simulink model "Free_Flight_PID_RPY_ARDrone_TrayZ"  (R2016b)
settings: configuration reference "AR_Drone_ConfigSet" (kept outside this file)
undefined symbols (not defined in the file): accelerometerXyzGains, accelerometerXyzOffsets, DiscIntNeverNeededParam, gyroXyzOffsets, Mag_Calib_Gain_Vector, Mag_Calib_Offset_Vector
libraries: simulink x6, AR_Drone_Sensors x2, AR_Drone_Actuators x2, vrlib x2, dspnetwork x1, simulink_extras x1, etargetslib x1
settings Model: DataDictionary=ArDroneDataDictionary.sldd  SimulationMode=external  ExtModeTrigDuration=48000  Creator=nraman  LastModifiedBy=SCBR
settings ConfigSetRef: DDName=ArDroneDataDictionary.sldd

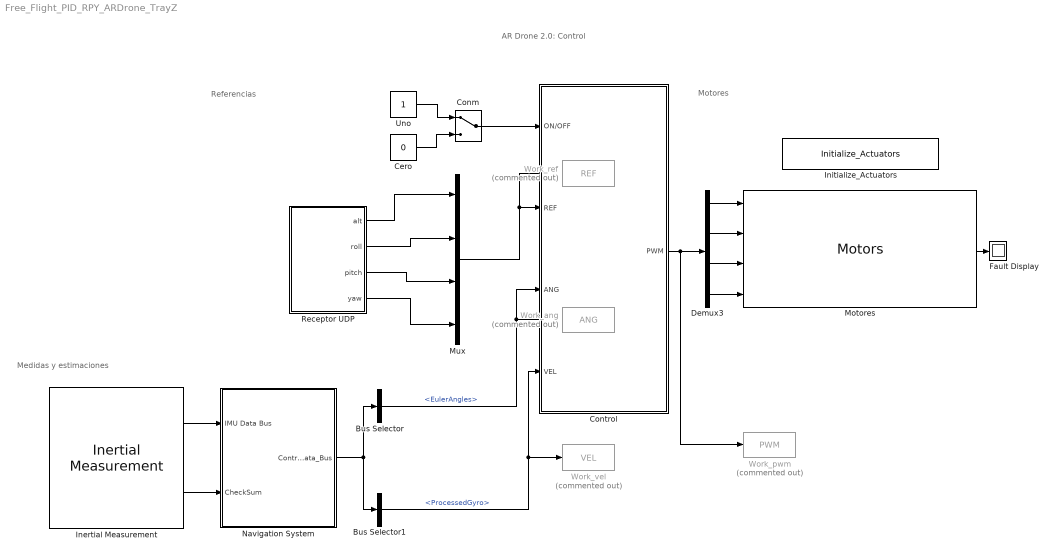
== system Free_Flight_PID_RPY_ARDrone_TrayZ ==
  note: AR Drone 2.0: Control
  note: Motores
  note: Medidas y estimaciones
  note: Referencias
  Bus Selector : BusSelector  OutputSignals=EulerAngles
  Bus Selector1 : BusSelector  OutputSignals=ProcessedGyro
  Cero : Constant  Value=0
  Conm : ManualSwitch
  Control : Subsystem
  Demux3 : Demux
  Fault Display : Display
  Inertial Measurement : AR_Drone_Sensors/Inertial Measurement  Ts=1/400
  Initialize_Actuators : AR_Drone_Actuators/Initialize_Actuators  ShowSpec=on
  Motores : AR_Drone_Actuators/Motors
  Mux : Mux
  Navigation System : Subsystem  AncestorBlock=AR_Drone_Positioning/Navigation System
  Receptor UDP : Subsystem
  Uno : Constant
  Work_ang : ToWorkspace  Commented=on  VariableName=ANG  SaveFormat=Structure With Time  SampleTime=0.0025
  Work_pwm : ToWorkspace  Commented=on  VariableName=PWM  SaveFormat=Structure With Time  SampleTime=0.0025
  Work_ref : ToWorkspace  Commented=on  VariableName=REF  SaveFormat=Structure With Time  SampleTime=0.0025
  Work_vel : ToWorkspace  Commented=on  VariableName=VEL  SaveFormat=Structure With Time  SampleTime=0.0025
  wires:
  Motores/1 -> Fault Display/1
  Demux3/1 -> Motores/1
  Demux3/2 -> Motores/2
  Demux3/3 -> Motores/3
  Demux3/4 -> Motores/4
  Inertial Measurement/1 -> Navigation System/1(IMU Data Bus)
  Inertial Measurement/2 -> Navigation System/2(CheckSum)
  Navigation System/1(Controller_Data_Bus) -> Bus Selector1/1, Bus Selector/1
  Bus Selector/1 -> Work_ang/1, Control/3(ANG)  "<EulerAngles>"
  Control/1(PWM) -> Work_pwm/1, Demux3/1
  Conm/1 -> Control/1(ON/OFF)
  Cero/1 -> Conm/2
  Uno/1 -> Conm/1
  Receptor UDP/1(alt) -> Mux/1
  Bus Selector1/1 -> Work_vel/1, Control/4(VEL)  "<ProcessedGyro>"
  Mux/1 -> Work_ref/1, Control/2(REF)
  Receptor UDP/2(roll) -> Mux/2
  Receptor UDP/3(pitch) -> Mux/3
  Receptor UDP/4(yaw) -> Mux/4

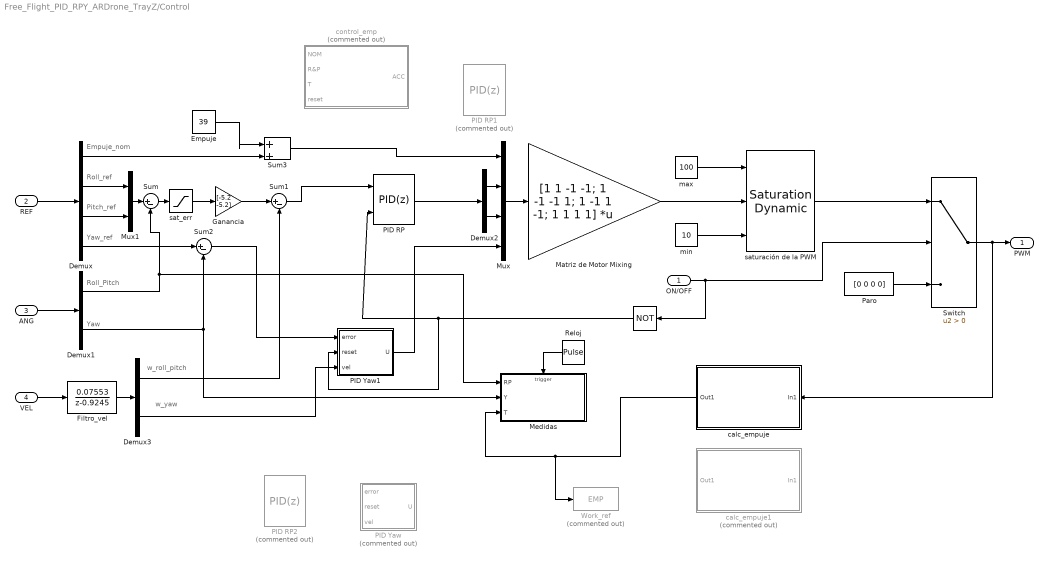
== system Free_Flight_PID_RPY_ARDrone_TrayZ/Control ==
  note: Empuje_nom
  note: Roll_ref
  note: Pitch_ref
  note: Yaw_ref
  note: Roll_Pitch
  note: Yaw
  note: w_roll_pitch
  note: w_yaw
  ON/OFF : Inport
  REF : Inport  Port=2
  ANG : Inport  Port=3
  VEL : Inport  Port=4
  " " : Logic  Operator=NOT  AllPortsSameDT=off  OutDataTypeStr=boolean
  Demux : Demux
  Demux1 : Demux  Outputs=[2 1]
  Demux2 : Demux  Outputs=2
  Demux3 : Demux  Outputs=[2 1]
  Empuje : Constant  Value=39
  Filtro_vel : DiscreteTransferFcn  Numerator=[0.07553]  Denominator=[1 -0.9245]
  Ganancia : Gain  Gain=[-5.2 -5.2]
  Matriz de Motor Mixing : Gain  Gain=[1 1 -1 -1; 1 -1 -1 1; 1 -1 1 -1; 1 1 1 1]  Multiplication=Matrix(K*u)  ParamDataTypeStr=int16  OutDataTypeStr=int16
  Medidas : Subsystem
  Mux : Mux
  Mux1 : Mux  Inputs=2
  PID RP : simulink/Continuous/PID Controller  Controller=PID  TimeDomain=Discrete-time  SampleTime=-1  IntegratorMethod=Forward Euler  FilterMethod=Forward Euler  Form=Parallel  UseFilter=on  ControllerParametersSource=internal  P=0.5  I=0.3  D=-0.04  N=5  InitialConditionSource=internal  InitialConditionForIntegrator=0  InitialConditionForFilter=0  ExternalReset=level  LimitOutput=on  UpperSaturationLimit=30  LowerSaturationLimit=-30  LinearizeAsGain=on  AntiWindupMode=clamping  Kb=1  TrackingMode=off  Kt=1  PParamMin=[]  PParamMax=[]  IParamMin=[]  IParamMax=[]  DParamMin=[]  DParamMax=[]  NParamMin=[]  NParamMax=[]  KbParamMin=[]  KbParamMax=[]  KtParamMin=[]  KtParamMax=[]  POutMin=[]  POutMax=[]  IOutMin=[]  IOutMax=[]  DOutMin=[]  DOutMax=[]  NOutMin=[]  NOutMax=[]  KbOutMin=[]  KbOutMax=[]  KtOutMin=[]  KtOutMax=[]  IntegratorOutMin=[]  IntegratorOutMax=[]  FilterOutMin=[]  FilterOutMax=[]  SumOutMin=[]  SumOutMax=[]  SumI1OutMin=[]  SumI1OutMax=[]  SumI2OutMin=[]  SumI2OutMax=[]  SumI3OutMin=[]  SumI3OutMax=[]  SumDOutMin=[]  SumDOutMax=[]  SaturationOutMin=[]  SaturationOutMax=[]  IntegratorContinuousStateAttributes=''  IntegratorStateMustResolveToSignalObject=off  IntegratorRTWStateStorageClass=Auto  FilterContinuousStateAttributes=''  FilterStateMustResolveToSignalObject=off  FilterRTWStateStorageClass=Auto  DifferentiatorICPrevScaledInput=0  DifferentiatorOutMin=[]  DifferentiatorOutMax=[]
  PID RP1 : simulink/Continuous/PID Controller  Commented=on  Controller=PID  TimeDomain=Discrete-time  SampleTime=-1  IntegratorMethod=Forward Euler  FilterMethod=Forward Euler  Form=Parallel  UseFilter=on  ControllerParametersSource=internal  P=0.45  I=0.25  D=-0.03  N=5  InitialConditionSource=internal  InitialConditionForIntegrator=0  InitialConditionForFilter=0  ExternalReset=level  LimitOutput=on  UpperSaturationLimit=30  LowerSaturationLimit=-30  LinearizeAsGain=on  AntiWindupMode=clamping  Kb=1  TrackingMode=off  Kt=1  PParamMin=[]  PParamMax=[]  IParamMin=[]  IParamMax=[]  DParamMin=[]  DParamMax=[]  NParamMin=[]  NParamMax=[]  KbParamMin=[]  KbParamMax=[]  KtParamMin=[]  KtParamMax=[]  POutMin=[]  POutMax=[]  IOutMin=[]  IOutMax=[]  DOutMin=[]  DOutMax=[]  NOutMin=[]  NOutMax=[]  KbOutMin=[]  KbOutMax=[]  KtOutMin=[]  KtOutMax=[]  IntegratorOutMin=[]  IntegratorOutMax=[]  FilterOutMin=[]  FilterOutMax=[]  SumOutMin=[]  SumOutMax=[]  SumI1OutMin=[]  SumI1OutMax=[]  SumI2OutMin=[]  SumI2OutMax=[]  SumI3OutMin=[]  SumI3OutMax=[]  SumDOutMin=[]  SumDOutMax=[]  SaturationOutMin=[]  SaturationOutMax=[]  IntegratorContinuousStateAttributes=''  IntegratorStateMustResolveToSignalObject=off  IntegratorRTWStateStorageClass=Auto  FilterContinuousStateAttributes=''  FilterStateMustResolveToSignalObject=off  FilterRTWStateStorageClass=Auto  DifferentiatorICPrevScaledInput=0  DifferentiatorOutMin=[]  DifferentiatorOutMax=[]
  PID RP2 : simulink/Continuous/PID Controller  Commented=on  Controller=PID  TimeDomain=Discrete-time  SampleTime=-1  IntegratorMethod=Forward Euler  FilterMethod=Forward Euler  Form=Parallel  UseFilter=on  ControllerParametersSource=internal  P=0.4  I=0.25  D=-0.05  N=5  InitialConditionSource=internal  InitialConditionForIntegrator=0  InitialConditionForFilter=0  ExternalReset=level  LimitOutput=on  UpperSaturationLimit=30  LowerSaturationLimit=-30  LinearizeAsGain=on  AntiWindupMode=clamping  Kb=1  TrackingMode=off  Kt=1  PParamMin=[]  PParamMax=[]  IParamMin=[]  IParamMax=[]  DParamMin=[]  DParamMax=[]  NParamMin=[]  NParamMax=[]  KbParamMin=[]  KbParamMax=[]  KtParamMin=[]  KtParamMax=[]  POutMin=[]  POutMax=[]  IOutMin=[]  IOutMax=[]  DOutMin=[]  DOutMax=[]  NOutMin=[]  NOutMax=[]  KbOutMin=[]  KbOutMax=[]  KtOutMin=[]  KtOutMax=[]  IntegratorOutMin=[]  IntegratorOutMax=[]  FilterOutMin=[]  FilterOutMax=[]  SumOutMin=[]  SumOutMax=[]  SumI1OutMin=[]  SumI1OutMax=[]  SumI2OutMin=[]  SumI2OutMax=[]  SumI3OutMin=[]  SumI3OutMax=[]  SumDOutMin=[]  SumDOutMax=[]  SaturationOutMin=[]  SaturationOutMax=[]  IntegratorContinuousStateAttributes=''  IntegratorStateMustResolveToSignalObject=off  IntegratorRTWStateStorageClass=Auto  FilterContinuousStateAttributes=''  FilterStateMustResolveToSignalObject=off  FilterRTWStateStorageClass=Auto  DifferentiatorICPrevScaledInput=0  DifferentiatorOutMin=[]  DifferentiatorOutMax=[]
  PID Yaw : Subsystem  Commented=on
  PID Yaw1 : Subsystem
  Paro : Constant  Value=[0 0 0 0]  OutDataTypeStr=int16
  Reloj : DiscretePulseGenerator  PulseType=Time based  Period=0.1  PulseWidth=50
  Sum : Sum  Inputs=|+-
  Sum1 : Sum  Inputs=|+-
  Sum2 : Sum  Inputs=|+-
  Sum3 : Sum  Inputs=|++
  Switch : Switch  Criteria=u2 > Threshold
  Work_ref : ToWorkspace  Commented=on  VariableName=EMP  SaveFormat=Structure With Time  SampleTime=0.0025
  calc_empuje : Subsystem
  calc_empuje1 : Subsystem  Commented=on
  control_emp : Subsystem  Commented=on
  max : Constant  Value=100  OutDataTypeStr=int16  SampleTime=-1
  min : Constant  Value=10  OutDataTypeStr=int16
  sat_err : Saturate  UpperLimit=[20 20]  LowerLimit=[-20 -20]
  saturación de la PWM : simulink/Discontinuities/Saturation Dynamic  OutMin=[]  OutMax=[]  OutDataTypeStr=Inherit: Same as second input  OutDataType=fixdt(1, 16)  OutScaling=2^-10  DoSatur=off
  PWM : Outport
  wires:
  Matriz de Motor Mixing/1 -> saturación de la PWM/2
  Paro/1 -> Switch/3
  ON/OFF/1 -> " "/1, Switch/2
  saturación de la PWM/1 -> Switch/1
  Mux/1 -> Matriz de Motor Mixing/1
  Switch/1 -> calc_empuje/1(In1), PWM/1
  min/1 -> saturación de la PWM/3
  max/1 -> saturación de la PWM/1
  ANG/1 -> Demux1/1
  VEL/1 -> Filtro_vel/1
  PID Yaw1/1(U) -> Mux/4
  Demux/2 -> Mux1/1
  Demux/3 -> Mux1/2
  Mux1/1 -> Sum/1
  Demux1/1 -> Sum/2, Medidas/1(RP)
  Demux/4 -> Sum2/1
  sat_err/1 -> Ganancia/1
  Demux2/1 -> Mux/2
  Demux2/2 -> Mux/3
  Ganancia/1 -> Sum1/1
  Sum1/1 -> PID RP/1
  Sum/1 -> sat_err/1
  " "/1 -> PID Yaw1/2(reset), PID RP/2
  PID RP/1 -> Demux2/1
  Demux3/1 -> Sum1/2
  Demux1/2 -> Medidas/2(Y), Sum2/2
  Sum2/1 -> PID Yaw1/1(error)
  Demux3/2 -> PID Yaw1/3(vel)
  Reloj/1 -> Medidas/Trigger
  calc_empuje/1(Out1) -> Work_ref/1, Medidas/3(T)
  Filtro_vel/1 -> Demux3/1
  REF/1 -> Demux/1
  Demux/1 -> Sum3/2
  Sum3/1 -> Mux/1
  Empuje/1 -> Sum3/1

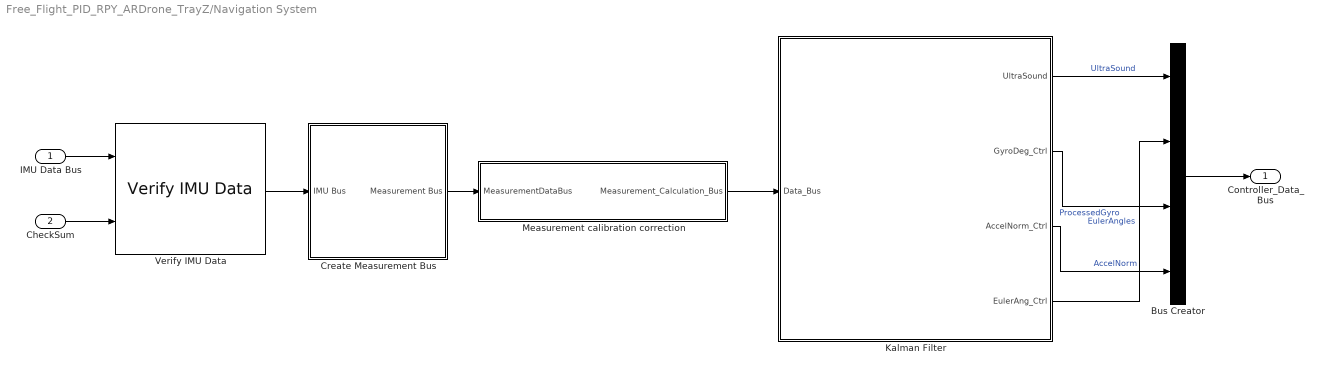
== system Free_Flight_PID_RPY_ARDrone_TrayZ/Navigation System ==
  IMU Data Bus : Inport  OutDataTypeStr=Bus: IMU_Packets
  CheckSum : Inport  Port=2
  Bus Creator : BusCreator  Inputs=4
  Create Measurement Bus : Subsystem
  Kalman Filter : Subsystem
  Measurement calibration correction : Subsystem
  Verify IMU Data : AR_Drone_Sensors/Verify IMU Data
  Controller_Data_Bus : Outport
  wires:
  Create Measurement Bus/1(Measurement Bus) -> Measurement calibration correction/1(MeasurementDataBus)
  Verify IMU Data/1 -> Create Measurement Bus/1(IMU Bus)
  Kalman Filter/3(AccelNorm_Ctrl) -> Bus Creator/4  "AccelNorm"
  Measurement calibration correction/1(Measurement_Calculation_Bus) -> Kalman Filter/1(Data_Bus)
  Bus Creator/1 -> Controller_Data_Bus/1
  Kalman Filter/1(UltraSound) -> Bus Creator/1  "UltraSound"
  Kalman Filter/2(GyroDeg_Ctrl) -> Bus Creator/3  "ProcessedGyro"
  CheckSum/1 -> Verify IMU Data/2
  Kalman Filter/4(EulerAng_Ctrl) -> Bus Creator/2  "EulerAngles"
  IMU Data Bus/1 -> Verify IMU Data/1

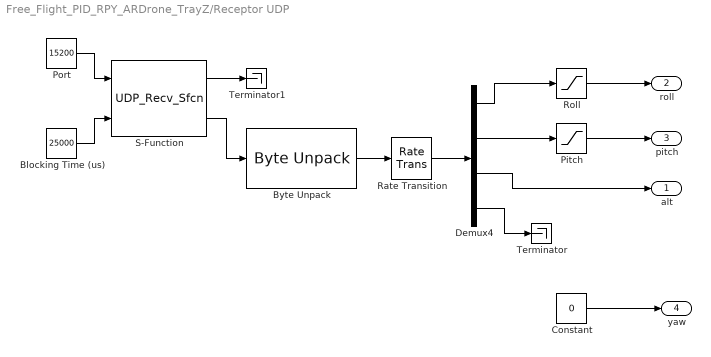
== system Free_Flight_PID_RPY_ARDrone_TrayZ/Receptor UDP ==
  Blocking Time (us) : Constant  Value=25000  OutDataTypeStr=double
  Byte Unpack : etargetslib/Byte Unpack  dimensions={[4]}  datatypes={'double'}  byteAlign=1
  Constant : Constant  Value=0
  Demux4 : Demux  Outputs=[1 1 1 1]
  Pitch : Saturate  UpperLimit=15  LowerLimit=-15
  Port : Constant  Value=15200  OutDataTypeStr=int32
  Rate Transition : RateTransition
  Roll : Saturate  UpperLimit=15  LowerLimit=-15
  S-Function : S-Function  FunctionName=UDP_Recv_Sfcn  Parameters=0.05  SFunctionDeploymentMode=off  EnableBusSupport=off
  Terminator : Terminator
  Terminator1 : Terminator
  alt : Outport
  roll : Outport  Port=2
  pitch : Outport  Port=3
  yaw : Outport  Port=4
  wires:
  Blocking Time (us)/1 -> S-Function/2
  S-Function/2 -> Byte Unpack/1
  Demux4/2 -> Pitch/1
  Demux4/1 -> Roll/1
  S-Function/1 -> Terminator1/1
  Byte Unpack/1 -> Rate Transition/1
  Port/1 -> S-Function/1
  Roll/1 -> roll/1
  Pitch/1 -> pitch/1
  Rate Transition/1 -> Demux4/1
  Constant/1 -> yaw/1
  Demux4/3 -> alt/1
  Demux4/4 -> Terminator/1

== system Free_Flight_PID_RPY_ARDrone_TrayZ/Control/Medidas ==
  RP : Inport
  Y : Inport  Port=2
  T : Inport  Port=3
  Trigger : TriggerPort  VariantControl=Variant  PortDimensions=1
  Mux : Mux  Inputs=3
  UDP Send : dspnetwork/UDP Send  remoteURL='192.168.1.2'  remotePort=50000  localURL='0.0.0.0'  localPortSource=Automatically determine  localPort=-1  sampletime=-1  blockPlatform=HOST  separateLengthPort=0
  wires:
  RP/1 -> Mux/1
  Mux/1 -> UDP Send/1
  T/1 -> Mux/3
  Y/1 -> Mux/2

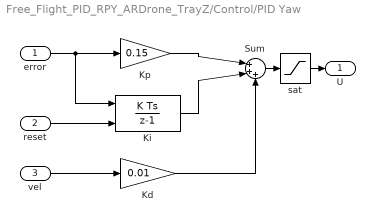
== system Free_Flight_PID_RPY_ARDrone_TrayZ/Control/PID Yaw ==
  error : Inport
  reset : Inport  Port=2
  vel : Inport  Port=3
  Kd : Gain  Gain=0.01
  Ki : DiscreteIntegrator  gainval=0.1  ExternalReset=level  InitialConditionSetting=State (most efficient)  SampleTime=-1  LimitOutput=on  UpperSaturationLimit=10  LowerSaturationLimit=-10  ICPrevOutput=DiscIntNeverNeededParam  ICPrevScaledInput=DiscIntNeverNeededParam
  Kp : Gain  Gain=0.15
  Sum : Sum  Inputs=|+++
  sat : Saturate  UpperLimit=20  LowerLimit=-20
  U : Outport
  wires:
  error/1 -> Ki/1, Kp/1
  Ki/1 -> Sum/2
  reset/1 -> Ki/2
  vel/1 -> Kd/1
  Kd/1 -> Sum/3
  Kp/1 -> Sum/1
  Sum/1 -> sat/1
  sat/1 -> U/1

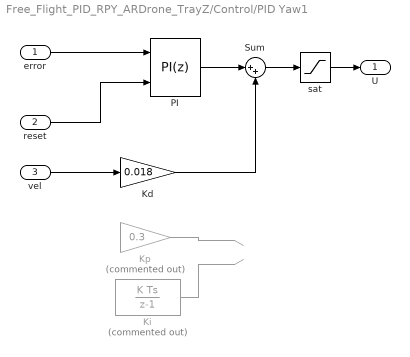
== system Free_Flight_PID_RPY_ARDrone_TrayZ/Control/PID Yaw1 ==
  error : Inport
  reset : Inport  Port=2
  vel : Inport  Port=3
  Kd : Gain  Gain=0.018
  Ki : DiscreteIntegrator  Commented=on  gainval=0.3  ExternalReset=level  InitialConditionSetting=State (most efficient)  SampleTime=-1  LimitOutput=on  UpperSaturationLimit=10  LowerSaturationLimit=-10  ICPrevOutput=DiscIntNeverNeededParam  ICPrevScaledInput=DiscIntNeverNeededParam
  Kp : Gain  Commented=on  Gain=0.3
  PI : simulink/Continuous/PID Controller  Controller=PI  TimeDomain=Discrete-time  SampleTime=-1  IntegratorMethod=Forward Euler  FilterMethod=Forward Euler  Form=Parallel  UseFilter=on  ControllerParametersSource=internal  P=0.25  I=0.25  D=-0.05  N=5  InitialConditionSource=internal  InitialConditionForIntegrator=0  InitialConditionForFilter=0  ExternalReset=level  LimitOutput=on  UpperSaturationLimit=20  LowerSaturationLimit=-20  LinearizeAsGain=on  AntiWindupMode=clamping  Kb=1  TrackingMode=off  Kt=1  PParamMin=[]  PParamMax=[]  IParamMin=[]  IParamMax=[]  DParamMin=[]  DParamMax=[]  NParamMin=[]  NParamMax=[]  KbParamMin=[]  KbParamMax=[]  KtParamMin=[]  KtParamMax=[]  POutMin=[]  POutMax=[]  IOutMin=[]  IOutMax=[]  DOutMin=[]  DOutMax=[]  NOutMin=[]  NOutMax=[]  KbOutMin=[]  KbOutMax=[]  KtOutMin=[]  KtOutMax=[]  IntegratorOutMin=[]  IntegratorOutMax=[]  FilterOutMin=[]  FilterOutMax=[]  SumOutMin=[]  SumOutMax=[]  SumI1OutMin=[]  SumI1OutMax=[]  SumI2OutMin=[]  SumI2OutMax=[]  SumI3OutMin=[]  SumI3OutMax=[]  SumDOutMin=[]  SumDOutMax=[]  SaturationOutMin=[]  SaturationOutMax=[]  IntegratorContinuousStateAttributes=''  IntegratorStateMustResolveToSignalObject=off  IntegratorRTWStateStorageClass=Auto  FilterContinuousStateAttributes=''  FilterStateMustResolveToSignalObject=off  FilterRTWStateStorageClass=Auto  DifferentiatorICPrevScaledInput=0  DifferentiatorOutMin=[]  DifferentiatorOutMax=[]
  Sum : Sum  Inputs=|++
  sat : Saturate  UpperLimit=20  LowerLimit=-20
  U : Outport
  wires:
  error/1 -> PI/1
  reset/1 -> PI/2
  vel/1 -> Kd/1
  Kd/1 -> Sum/2
  Sum/1 -> sat/1
  sat/1 -> U/1
  Ki/1 -> ?
  Kp/1 -> ?
  PI/1 -> Sum/1

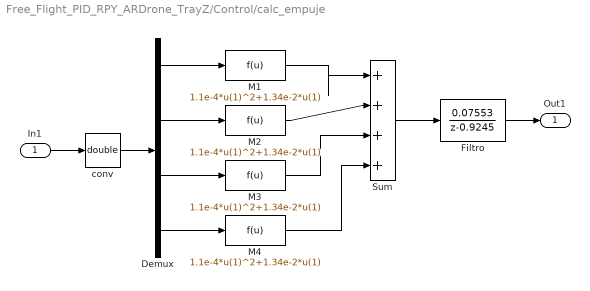
== system Free_Flight_PID_RPY_ARDrone_TrayZ/Control/calc_empuje ==
  In1 : Inport
  Demux : Demux
  Filtro : DiscreteTransferFcn  Numerator=[0.07553]  Denominator=[1 -0.9245]
  M{1..4} (4 alike) : Fcn  Expr=1.1e-4*u(1)^2+1.34e-2*u(1)
  Sum : Sum  Inputs=|++++
  conv : DataTypeConversion  OutDataTypeStr=double  RndMeth=Nearest
  Out1 : Outport
  wires:
  Demux/1 -> M1/1
  Demux/2 -> M2/1
  Demux/3 -> M3/1
  Demux/4 -> M4/1
  M1/1 -> Sum/1
  M2/1 -> Sum/2
  M3/1 -> Sum/3
  M4/1 -> Sum/4
  conv/1 -> Demux/1
  In1/1 -> conv/1
  Filtro/1 -> Out1/1
  Sum/1 -> Filtro/1

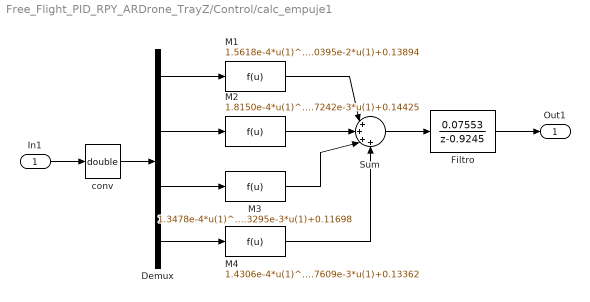
== system Free_Flight_PID_RPY_ARDrone_TrayZ/Control/calc_empuje1 ==
  In1 : Inport
  Demux : Demux
  Filtro : DiscreteTransferFcn  Numerator=[0.07553]  Denominator=[1 -0.9245]
  M1 : Fcn  Expr=1.5618e-4*u(1)^2+1.0395e-2*u(1)+0.13894
  M2 : Fcn  Expr=1.8150e-4*u(1)^2+8.7242e-3*u(1)+0.14425
  M3 : Fcn  Expr=1.3478e-4*u(1)^2+7.3295e-3*u(1)+0.11698
  M4 : Fcn  Expr=1.4306e-4*u(1)^2+5.7609e-3*u(1)+0.13362
  Sum : Sum  Inputs=|++++
  conv : DataTypeConversion  OutDataTypeStr=double  RndMeth=Nearest
  Out1 : Outport
  wires:
  Demux/1 -> M1/1
  Demux/2 -> M2/1
  Demux/3 -> M3/1
  Demux/4 -> M4/1
  M1/1 -> Sum/1
  M2/1 -> Sum/2
  M3/1 -> Sum/3
  M4/1 -> Sum/4
  conv/1 -> Demux/1
  In1/1 -> conv/1
  Filtro/1 -> Out1/1
  Sum/1 -> Filtro/1

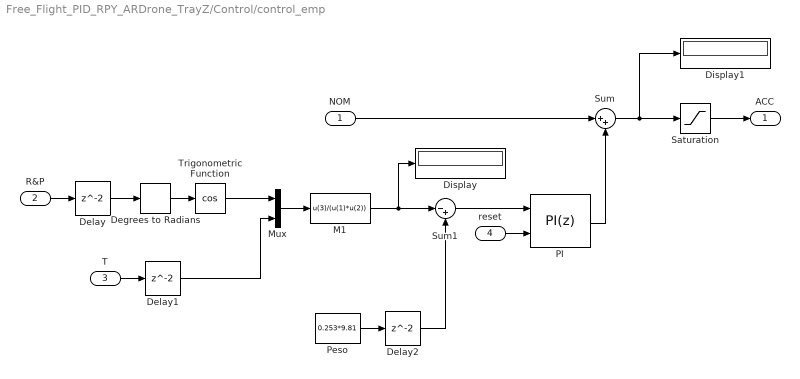
== system Free_Flight_PID_RPY_ARDrone_TrayZ/Control/control_emp ==
  NOM : Inport
  R&P : Inport  Port=2
  T : Inport  Port=3
  reset : Inport  Port=4
  Degrees to Radians : simulink_extras/Transformations/Degrees to Radians
  Delay : Delay
  Delay1 : Delay
  Delay2 : Delay
  Display : Display
  Display1 : Display
  M1 : Fcn  Expr=u(3)/(u(1)*u(2))
  Mux : Mux  Inputs=2
  PI : simulink/Continuous/PID Controller  Controller=PI  TimeDomain=Discrete-time  SampleTime=-1  IntegratorMethod=Forward Euler  FilterMethod=Forward Euler  Form=Parallel  UseFilter=on  ControllerParametersSource=internal  P=15  I=3  D=-0.05  N=5  InitialConditionSource=internal  InitialConditionForIntegrator=0  InitialConditionForFilter=0  ExternalReset=level  LimitOutput=on  UpperSaturationLimit=20  LowerSaturationLimit=-20  LinearizeAsGain=on  AntiWindupMode=clamping  Kb=1  TrackingMode=off  Kt=1  PParamMin=[]  PParamMax=[]  IParamMin=[]  IParamMax=[]  DParamMin=[]  DParamMax=[]  NParamMin=[]  NParamMax=[]  KbParamMin=[]  KbParamMax=[]  KtParamMin=[]  KtParamMax=[]  POutMin=[]  POutMax=[]  IOutMin=[]  IOutMax=[]  DOutMin=[]  DOutMax=[]  NOutMin=[]  NOutMax=[]  KbOutMin=[]  KbOutMax=[]  KtOutMin=[]  KtOutMax=[]  IntegratorOutMin=[]  IntegratorOutMax=[]  FilterOutMin=[]  FilterOutMax=[]  SumOutMin=[]  SumOutMax=[]  SumI1OutMin=[]  SumI1OutMax=[]  SumI2OutMin=[]  SumI2OutMax=[]  SumI3OutMin=[]  SumI3OutMax=[]  SumDOutMin=[]  SumDOutMax=[]  SaturationOutMin=[]  SaturationOutMax=[]  IntegratorContinuousStateAttributes=''  IntegratorStateMustResolveToSignalObject=off  IntegratorRTWStateStorageClass=Auto  FilterContinuousStateAttributes=''  FilterStateMustResolveToSignalObject=off  FilterRTWStateStorageClass=Auto  DifferentiatorICPrevScaledInput=0  DifferentiatorOutMin=[]  DifferentiatorOutMax=[]
  Peso : Constant  Value=0.253*9.81
  Saturation : Saturate  UpperLimit=60  LowerLimit=10
  Sum : Sum  Inputs=|++
  Sum1 : Sum  Inputs=|-+
  Trigonometric Function : Trigonometry  Operator=cos
  ACC : Outport
  wires:
  Sum/1 -> Display1/1, Saturation/1
  NOM/1 -> Sum/1
  Peso/1 -> Delay2/1
  Sum1/1 -> PI/1
  PI/1 -> Sum/2
  reset/1 -> PI/2
  R&P/1 -> Delay/1
  Degrees to Radians/1 -> Trigonometric Function/1
  Mux/1 -> M1/1
  T/1 -> Delay1/1
  M1/1 -> Display/1, Sum1/1
  Delay1/1 -> Mux/2
  Delay/1 -> Degrees to Radians/1
  Delay2/1 -> Sum1/2
  Trigonometric Function/1 -> Mux/1
  Saturation/1 -> ACC/1

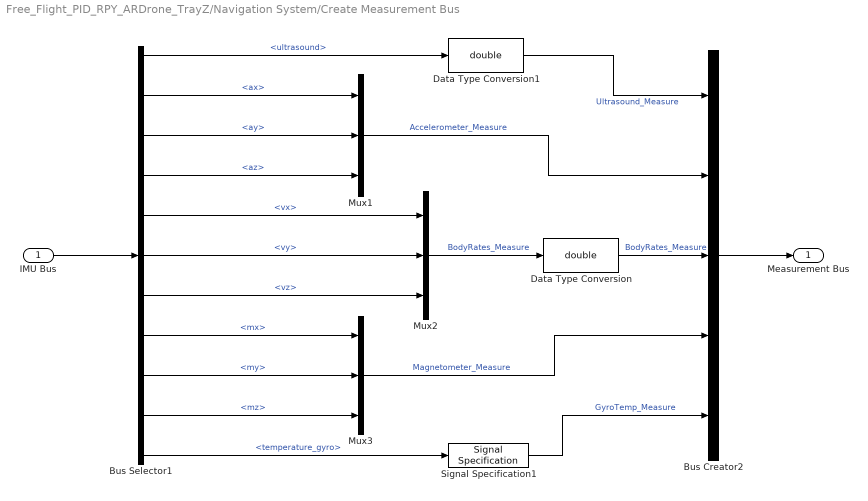
== system Free_Flight_PID_RPY_ARDrone_TrayZ/Navigation System/Create Measurement Bus ==
  IMU Bus : Inport
  Bus Creator2 : BusCreator  Inputs=5
  Bus Selector1 : BusSelector  OutputSignals=ultrasound,ax,ay,az,vx,vy,vz,mx,my,mz,temperature_gyro
  Data Type Conversion : DataTypeConversion  OutDataTypeStr=double
  Data Type Conversion1 : DataTypeConversion  OutDataTypeStr=double
  Mux1 : Mux  Inputs=3
  Mux2 : Mux  Inputs=3
  Mux3 : Mux  Inputs=3
  Signal Specification1 : SignalSpecification
  Measurement Bus : Outport
  wires:
  Mux1/1 -> Bus Creator2/2  "Accelerometer_Measure"
  Bus Selector1/2 -> Mux1/1  "<ax>"
  Mux3/1 -> Bus Creator2/4  "Magnetometer_Measure"
  Data Type Conversion/1 -> Bus Creator2/3  "BodyRates_Measure"
  Bus Selector1/3 -> Mux1/2  "<ay>"
  Signal Specification1/1 -> Bus Creator2/5  "GyroTemp_Measure"
  Bus Selector1/4 -> Mux1/3  "<az>"
  Bus Selector1/9 -> Mux3/2  "<my>"
  Bus Selector1/10 -> Mux3/3  "<mz>"
  Bus Selector1/8 -> Mux3/1  "<mx>"
  IMU Bus/1 -> Bus Selector1/1
  Bus Selector1/5 -> Mux2/1  "<vx>"
  Bus Selector1/7 -> Mux2/3  "<vz>"
  Bus Selector1/6 -> Mux2/2  "<vy>"
  Bus Selector1/1 -> Data Type Conversion1/1  "<ultrasound>"
  Bus Selector1/11 -> Signal Specification1/1  "<temperature_gyro>"
  Data Type Conversion1/1 -> Bus Creator2/1  "Ultrasound_Measure"
  Bus Creator2/1 -> Measurement Bus/1
  Mux2/1 -> Data Type Conversion/1  "BodyRates_Measure"

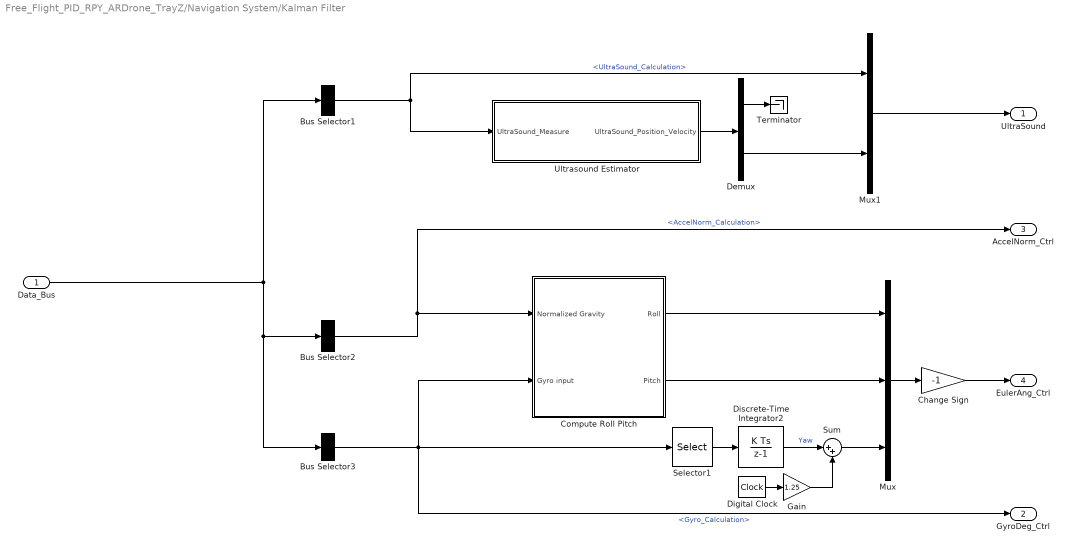
== system Free_Flight_PID_RPY_ARDrone_TrayZ/Navigation System/Kalman Filter ==
  Data_Bus : Inport
  Bus Selector1 : BusSelector  OutputSignals=UltraSound_Calculation
  Bus Selector2 : BusSelector  OutputSignals=AccelNorm_Calculation
  Bus Selector3 : BusSelector  OutputSignals=Gyro_Calculation
  Change Sign : Gain  Gain=-1
  Compute Roll Pitch : Subsystem
  Demux : Demux  Outputs=2
  Digital Clock : DigitalClock  SampleTime=1/400
  Discrete-Time Integrator2 : DiscreteIntegrator  SampleTime=-1  OutDataTypeStr=double  ICPrevOutput=DiscIntNeverNeededParam  ICPrevScaledInput=DiscIntNeverNeededParam
  Gain : Gain  Gain=1.25
  Mux : Mux  Inputs=3
  Mux1 : Mux  Inputs=2
  Selector1 : Selector  IndexMode=Zero-based  InputPortWidth=3  IndexOptions=Index vector (dialog)  Indices=[2]  OutputSizes=1
  Sum : Sum  Inputs=|++
  Terminator : Terminator
  Ultrasound Estimator : Subsystem
  UltraSound : Outport
  GyroDeg_Ctrl : Outport  Port=2
  AccelNorm_Ctrl : Outport  Port=3
  EulerAng_Ctrl : Outport  Port=4
  wires:
  Compute Roll Pitch/2(Pitch) -> Mux/2
  Compute Roll Pitch/1(Roll) -> Mux/1
  Selector1/1 -> Discrete-Time Integrator2/1
  Demux/1 -> Terminator/1
  Mux1/1 -> UltraSound/1
  Demux/2 -> Mux1/2
  Change Sign/1 -> EulerAng_Ctrl/1
  Ultrasound Estimator/1("UltraSound_Position_Velocity ") -> Demux/1
  Bus Selector2/1 -> Compute Roll Pitch/1(Normalized Gravity), AccelNorm_Ctrl/1  "<AccelNorm_Calculation>"
  Mux/1 -> Change Sign/1
  Bus Selector3/1 -> GyroDeg_Ctrl/1, Selector1/1, Compute Roll Pitch/2(Gyro input)  "<Gyro_Calculation>"
  Data_Bus/1 -> Bus Selector1/1, Bus Selector2/1, Bus Selector3/1
  Bus Selector1/1 -> Ultrasound Estimator/1(UltraSound_Measure), Mux1/1  "<UltraSound_Calculation>"
  Discrete-Time Integrator2/1 -> Sum/1  "Yaw"
  Sum/1 -> Mux/3
  Digital Clock/1 -> Gain/1
  Gain/1 -> Sum/2

== system Free_Flight_PID_RPY_ARDrone_TrayZ/Navigation System/Measurement calibration correction ==
  MeasurementDataBus : Inport
  Accelerometer calibration : Subsystem
  Bus Creator1 : BusCreator  Inputs=4
  Bus Selector : BusSelector  OutputSignals=Ultrasound_Measure,Accelerometer_Measure,BodyRates_Measure,Magnetometer_Measure
  Calibration_Scale_and_Offset : Subsystem
  Gyro offset : Subsystem
  MATLAB Function : MATLAB Function  TreatAsAtomicUnit=on
  Measurement_Calculation_Bus : Outport
  wires:
  Bus Selector/1 -> MATLAB Function/1(Ultrasound_Measure)  "<Ultrasound_Measure>"
  Gyro offset/1(Gyro Offset Remove) -> Bus Creator1/3  "Gyro_Calculation"
  Bus Selector/2 -> Accelerometer calibration/1(Accel)  "<Accelerometer_Measure>"
  Accelerometer calibration/1(Accel_Norm) -> Bus Creator1/2  "AccelNorm_Calculation"
  MATLAB Function/1(UltraSound_Calculation) -> Bus Creator1/1  "UltraSound_Calculation"
  Calibration_Scale_and_Offset/1(Normalized  Magnetometer) -> Bus Creator1/4  "Magnetometer_Calculation"
  MeasurementDataBus/1 -> Bus Selector/1
  Bus Selector/3 -> Gyro offset/1(Raw Gyro Values)  "<BodyRates_Measure>"
  Bus Creator1/1 -> Measurement_Calculation_Bus/1
  Bus Selector/4 -> Calibration_Scale_and_Offset/1(RawMag)  "<Magnetometer_Measure>"

== system Free_Flight_PID_RPY_ARDrone_TrayZ/Navigation System/Kalman Filter/Compute Roll Pitch ==
  Normalized Gravity : Inport
  Gyro input : Inport  Port=2
  Calculate Roll - Pitch : Subsystem
  KF_PITCH : Subsystem
  KF_ROLL : Subsystem
  Seperate Data : Subsystem
  Roll : Outport
  Pitch : Outport  Port=2
  wires:
  Seperate Data/1(Gyro_Roll_Ctrl) -> KF_ROLL/2(GYRO_ROLL_CTRL_IN)
  Seperate Data/2(Gyro_Pitch_Ctrl) -> KF_PITCH/1(GYRO_CTRL_IN)
  Calculate Roll - Pitch/1(RollRaw) -> KF_ROLL/1(ROLL_ACCEL_MEASURE)
  KF_ROLL/1(ROLL_FILTERED) -> Roll/1
  KF_PITCH/1(PITCH_FILTERED) -> Pitch/1  "Pitch"
  Calculate Roll - Pitch/2(PitchRaw) -> KF_PITCH/2(PITCH_ACCEL_MEASURE)
  Gyro input/1 -> Seperate Data/1(GyroIn)
  Normalized Gravity/1 -> Calculate Roll - Pitch/1(Normalized Gravity Vector)

== system Free_Flight_PID_RPY_ARDrone_TrayZ/Navigation System/Kalman Filter/Ultrasound Estimator ==
  UltraSound_Measure : Inport
  Kalman Tracker : MATLAB Function  TreatAsAtomicUnit=on
  Unit Delay1 : UnitDelay  InitialCondition=[0 0 ]  SampleTime=-1
  Unit Delay2 : UnitDelay  InitialCondition=eye(2)  SampleTime=-1
  "UltraSound_Position_Velocity " : Outport
  wires:
  Unit Delay1/1 -> Kalman Tracker/3(state_correction_input), "UltraSound_Position_Velocity "/1
  Unit Delay2/1 -> Kalman Tracker/2(covariance_correction_input)
  UltraSound_Measure/1 -> Kalman Tracker/1(UltraSoundMeasure)
  Kalman Tracker/1(state_correction) -> Unit Delay1/1
  Kalman Tracker/2(covariance_correction) -> Unit Delay2/1

== system Free_Flight_PID_RPY_ARDrone_TrayZ/Navigation System/Measurement calibration correction/Accelerometer calibration ==
  Accel : Inport
  Apply calibration parameters : Subsystem
  Data Type Conversion : DataTypeConversion  OutDataTypeStr=double
  Low pass filter : Subsystem
  Normalize Vector : vrlib/Utilities/Normalize Vector  maxzero=0
  Accel_Norm : Outport
  wires:
  Accel/1 -> Data Type Conversion/1
  Data Type Conversion/1 -> Apply calibration parameters/1(Raw Accelerometer Data)
  Apply calibration parameters/1(Calibrated Accelerometer Data) -> Low pass filter/1(Offset Accel)
  Low pass filter/1(Filtered Accel) -> Normalize Vector/1
  Normalize Vector/1 -> Accel_Norm/1

== system Free_Flight_PID_RPY_ARDrone_TrayZ/Navigation System/Measurement calibration correction/Calibration_Scale_and_Offset ==
  RawMag : Inport
  Normalize Vector : vrlib/Utilities/Normalize Vector  maxzero=0
  Process Magnetometer : Subsystem
  Normalized  Magnetometer : Outport
  wires:
  RawMag/1 -> Process Magnetometer/1(Magnetometer)
  Process Magnetometer/1(MagVector) -> Normalize Vector/1
  Normalize Vector/1 -> Normalized  Magnetometer/1

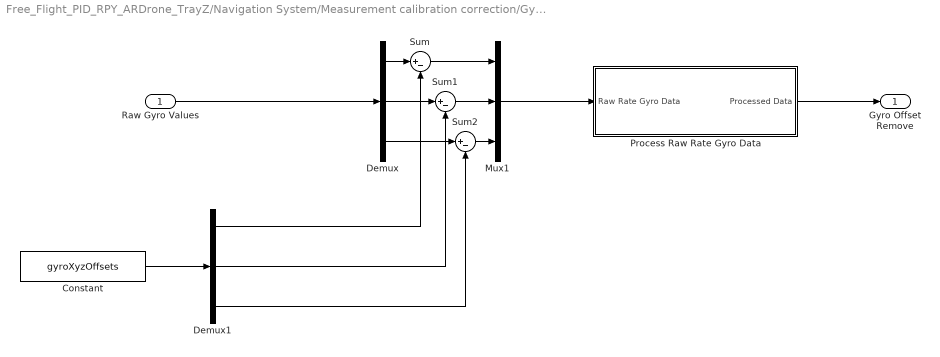
== system Free_Flight_PID_RPY_ARDrone_TrayZ/Navigation System/Measurement calibration correction/Gyro offset ==
  Raw Gyro Values : Inport
  Constant : Constant  Value=gyroXyzOffsets  VectorParams1D=off
  Demux : Demux  Outputs=3
  Demux1 : Demux  Outputs=3
  Mux1 : Mux  Inputs=3
  Process Raw Rate Gyro Data : Subsystem
  Sum : Sum  Inputs=|+-
  Sum1 : Sum  Inputs=|+-
  Sum2 : Sum  Inputs=|+-
  Gyro Offset Remove : Outport
  wires:
  Demux/3 -> Sum2/1
  Sum1/1 -> Mux1/2
  Demux1/1 -> Sum/2
  Sum2/1 -> Mux1/3
  Demux/2 -> Sum1/1
  Demux/1 -> Sum/1
  Sum/1 -> Mux1/1
  Mux1/1 -> Process Raw Rate Gyro Data/1(Raw Rate Gyro Data)
  Demux1/2 -> Sum1/2
  Demux1/3 -> Sum2/2
  Process Raw Rate Gyro Data/1(Processed Data) -> Gyro Offset Remove/1
  Constant/1 -> Demux1/1
  Raw Gyro Values/1 -> Demux/1

== system Free_Flight_PID_RPY_ARDrone_TrayZ/Navigation System/Kalman Filter/Compute Roll Pitch/Calculate Roll - Pitch ==
  note: http://www.digikey.com/en/articles/techzone/2011/may/using-an-accelerometer-for-inclination-sensing
  Normalized Gravity Vector : Inport
  Gain4 : Gain  Gain=180/pi
  Gain5 : Gain  Gain=-180/pi
  MATLAB Function : MATLAB Function  TreatAsAtomicUnit=on
  RollRaw : Outport
  PitchRaw : Outport  Port=2
  wires:
  Gain5/1 -> PitchRaw/1
  Gain4/1 -> RollRaw/1
  MATLAB Function/2(Pitch) -> Gain5/1  "roll"
  MATLAB Function/1(Roll) -> Gain4/1  "pitch"
  Normalized Gravity Vector/1 -> MATLAB Function/1(Ax_Ay_Az)

== system Free_Flight_PID_RPY_ARDrone_TrayZ/Navigation System/Kalman Filter/Compute Roll Pitch/KF_PITCH ==
  GYRO_CTRL_IN : Inport
  PITCH_ACCEL_MEASURE : Inport  Port=2
  Demux : Demux  Outputs=2
  Kalman Tracker : MATLAB Function  TreatAsAtomicUnit=on
  Terminator : Terminator
  Unit Delay : UnitDelay  InitialCondition=eye(2)  SampleTime=-1
  Unit Delay1 : UnitDelay  InitialCondition=[0 0]'  SampleTime=-1
  PITCH_FILTERED : Outport
  wires:
  Demux/2 -> Terminator/1  "B_dot"
  PITCH_ACCEL_MEASURE/1 -> Kalman Tracker/4(measurement_angle)
  Unit Delay/1 -> Kalman Tracker/2(covariance_correction_prev)
  GYRO_CTRL_IN/1 -> Kalman Tracker/3(ctrl_input_gyro)
  Unit Delay1/1 -> Kalman Tracker/1(prev_state)
  Kalman Tracker/1(state_correction) -> Demux/1, Unit Delay1/1
  Demux/1 -> PITCH_FILTERED/1
  Kalman Tracker/2(covariance_correction) -> Unit Delay/1

== system Free_Flight_PID_RPY_ARDrone_TrayZ/Navigation System/Kalman Filter/Compute Roll Pitch/KF_ROLL ==
  ROLL_ACCEL_MEASURE : Inport
  GYRO_ROLL_CTRL_IN : Inport  Port=2
  Demux : Demux  Outputs=2
  Kalman Tracker : MATLAB Function  TreatAsAtomicUnit=on
  Terminator : Terminator
  Unit Delay : UnitDelay  InitialCondition=eye(2)  SampleTime=-1
  Unit Delay1 : UnitDelay  InitialCondition=[0 0]'  SampleTime=-1
  ROLL_FILTERED : Outport
  wires:
  Demux/2 -> Terminator/1  "B_dot"
  Demux/1 -> ROLL_FILTERED/1
  ROLL_ACCEL_MEASURE/1 -> Kalman Tracker/4(measurement_angle)
  Unit Delay/1 -> Kalman Tracker/2(covariance_correction_prev)
  GYRO_ROLL_CTRL_IN/1 -> Kalman Tracker/3(ctrl_input_gyro)
  Unit Delay1/1 -> Kalman Tracker/1(prev_state)
  Kalman Tracker/1(state_correction) -> Demux/1, Unit Delay1/1
  Kalman Tracker/2(covariance_correction) -> Unit Delay/1

== system Free_Flight_PID_RPY_ARDrone_TrayZ/Navigation System/Kalman Filter/Compute Roll Pitch/Seperate Data ==
  GyroIn : Inport
  Demux1 : Demux  Outputs=[1 1]
  Selector2 : Selector  IndexMode=Zero-based  InputPortWidth=3  IndexOptions=Index vector (dialog)  Indices=[0 1]  OutputSizes=1
  Gyro_Roll_Ctrl : Outport
  Gyro_Pitch_Ctrl : Outport  Port=2
  wires:
  Selector2/1 -> Demux1/1
  Demux1/2 -> Gyro_Pitch_Ctrl/1  "GYRO_Y"
  Demux1/1 -> Gyro_Roll_Ctrl/1  "GYRO_X"
  GyroIn/1 -> Selector2/1

== system Free_Flight_PID_RPY_ARDrone_TrayZ/Navigation System/Measurement calibration correction/Accelerometer calibration/Apply calibration parameters ==
  Raw Accelerometer Data : Inport
  Acclerometer Calibration Gains : Constant  Value=accelerometerXyzGains
  Acclerometer Calibration Offsets : Constant  Value=accelerometerXyzOffsets
  Add : Sum  Inputs=+-
  Divide : Product  Inputs=*/
  Invert Axes Definition : Gain  Gain=-1
  Calibrated Accelerometer Data : Outport
  wires:
  Invert Axes Definition/1 -> Calibrated Accelerometer Data/1
  Raw Accelerometer Data/1 -> Add/1
  Acclerometer Calibration Gains/1 -> Divide/2
  Acclerometer Calibration Offsets/1 -> Add/2
  Divide/1 -> Invert Axes Definition/1
  Add/1 -> Divide/1

== system Free_Flight_PID_RPY_ARDrone_TrayZ/Navigation System/Measurement calibration correction/Accelerometer calibration/Low pass filter ==
  Offset Accel : Inport
  Add : Sum
  Gain : Gain  Gain=0.8
  Gain1 : Gain  Gain=0.2
  Unit Delay : UnitDelay  SampleTime=-1
  Filtered Accel : Outport
  wires:
  Unit Delay/1 -> Gain/1
  Add/1 -> Unit Delay/1, Filtered Accel/1
  Gain1/1 -> Add/1
  Gain/1 -> Add/2
  Offset Accel/1 -> Gain1/1

== system Free_Flight_PID_RPY_ARDrone_TrayZ/Navigation System/Measurement calibration correction/Calibration_Scale_and_Offset/Process Magnetometer ==
  note: magnetometer[ 0 ] = - ( float ) navdata.mx ;
      | magnetometer[ 1 ] = ( float ) navdata.my ;
      | magnetometer[ 2 ] = - ( float ) navdata.mz ;
      | const float Sensitivity[ 3 ] = { 0.0071492608 , 0.0070882491 , 0.0074057781 } ;
      | const float Neutral[ 3 ] = { 118.0 , - 65.0 , 110.0 } ;
  Magnetometer : Inport
  Constant : Constant  Value=[Mag_Calib_Offset_Vector.Gain_X Mag_Calib_Offset_Vector.Gain_Y Mag_Calib_Offset_Vector.Gain_Z]
      settings: AttributesFormatString=%<Value>
  Constant1 : Constant  Value=[Mag_Calib_Gain_Vector.Gain_X Mag_Calib_Gain_Vector.Gain_Y Mag_Calib_Gain_Vector.Gain_Z]
      settings: AttributesFormatString=%<Value>
  Divide : Product  Inputs=/*
  Sum : Sum  Inputs=|+-
  MagVector : Outport
  wires:
  Divide/1 -> MagVector/1
  Constant1/1 -> Divide/1
  Constant/1 -> Sum/2
  Magnetometer/1 -> Sum/1
  Sum/1 -> Divide/2

== system Free_Flight_PID_RPY_ARDrone_TrayZ/Navigation System/Measurement calibration correction/Gyro offset/Process Raw Rate Gyro Data ==
  note: const float Sensitivity[ 3 ] = { 0.0609 , 0.0609 , 0.0609 } ;
  Raw Rate Gyro Data : Inport
  Gain : Gain  Gain=[0.0609, 0.0609, 0.0609]  ParamDataTypeStr=double
  Processed Data : Outport
  wires:
  Raw Rate Gyro Data/1 -> Gain/1
  Gain/1 -> Processed Data/1

== matlab function Free_Flight_PID_RPY_ARDrone_TrayZ/Navigation System/Kalman Filter/Compute Roll Pitch/Calculate Roll - Pitch/MATLAB Function ==
  data: Ax_Ay_Az input; Roll output; Pitch output
function [Roll,Pitch] = CalculateAngle(Ax_Ay_Az)
%#codegen
Ax = -Ax_Ay_Az(1);
Ay = -Ax_Ay_Az(2);
Az = Ax_Ay_Az(3);

Pitch = atan( Ax / sqrt( Ay^2 + Az^2));
Roll = atan( Ay / sqrt( Ax^2 + Az^2));

== matlab function Free_Flight_PID_RPY_ARDrone_TrayZ/Navigation System/Measurement calibration correction/MATLAB Function ==
  data: Ultrasound_Measure input; UltraSound_Calculation output
function UltraSound_Calculation = removePeak(Ultrasound_Measure)
%#codegen

peakThreshold = 10000;

persistent validHeight
if isempty(validHeight)
    validHeight = 0;
end

if Ultrasound_Measure < peakThreshold
    validHeight = (Ultrasound_Measure - 880) / 26.533;
end

UltraSound_Calculation = validHeight;

== matlab function Free_Flight_PID_RPY_ARDrone_TrayZ/Navigation System/Kalman Filter/Compute Roll Pitch/KF_ROLL/Kalman Tracker ==
  data: prev_state input; covariance_correction_prev input; state_correction output; covariance_correction output; ctrl_input_gyro input; measurement_angle input
function [state_correction, covariance_correction] = fcn(prev_state, covariance_correction_prev, ctrl_input_gyro, measurement_angle)


%-------------------------------
%-------------------------------
%---- Predict Stage ------------
%-------------------------------
%-------------------------------
% pix_value = 5;
Ts = 1/400;
%Process Noise
p_var =0.01;
Q = [p_var^2     0         
      0         p_var^2];

%A matrix
A =  [1   -Ts 
      0   1];

%odutput these values with a unit delay (for algebraic loop), apply initial conditions
state_prediction = A*prev_state + [Ts 0; 0 0]*[ctrl_input_gyro; 0 ];
covariance_prediction = A*covariance_correction_prev*A' + Q;

%-------------------------------
%-------------------------------
%---- Estimate Stage -----------
%-------------------------------
%-------------------------------

    %H matrix
    H = [1 0];

    %Measurement noise from accelerometer angle measurement
    m_var = 0.5;
%     m_var_r = 1;

    R = [m_var^2 ];

    %Measurement Z
    Z = [measurement_angle];

    %Compute Kalman Gain
    Kalman_Gain = covariance_prediction*H'*inv(H*covariance_prediction*H'+R); %2x2 matrix

    %compute state space correction based on measurement
    state_correction = state_prediction + Kalman_Gain*(Z - H*state_prediction); %4x1 vector of states

    %compute covariance correction
    covariance_correction = (eye(2) - Kalman_Gain*H)*covariance_prediction; %2x2 covariance matrix

%     corrected_angle_measure = state_correction(1) - Ts*state_correction(2);
end

== matlab function Free_Flight_PID_RPY_ARDrone_TrayZ/Navigation System/Kalman Filter/Compute Roll Pitch/KF_PITCH/Kalman Tracker ==
  data: prev_state input; covariance_correction_prev input; state_correction output; covariance_correction output; ctrl_input_gyro input; measurement_angle input
function [state_correction, covariance_correction] = fcn(prev_state, covariance_correction_prev, ctrl_input_gyro, measurement_angle)


%-------------------------------
%-------------------------------
%---- Predict Stage ------------
%-------------------------------
%-------------------------------
% pix_value = 5;
Ts = 1/400;
%Process Noise
p_var =0.01;
Q = [p_var^2     0         
      0         p_var^2];

%A matrix
A =  [1   -Ts 
      0   1];

%odutput these values with a unit delay (for algebraic loop), apply initial conditions
state_prediction = A*prev_state + [Ts 0; 0 0]*[ctrl_input_gyro; 0 ];
covariance_prediction = A*covariance_correction_prev*A' + Q;

%-------------------------------
%-------------------------------
%---- Estimate Stage -----------
%-------------------------------
%-------------------------------

    %H matrix
    H = [1 0];

    %Measurement noise from accelerometer angle measurement
    m_var = 1;
%     m_var_r = 1;

    R = [m_var^2 ];

    %Measurement Z
    Z = [measurement_angle];

    %Compute Kalman Gain
    Kalman_Gain = covariance_prediction*H'*inv(H*covariance_prediction*H'+R); %2x2 matrix

    %compute state space correction based on measurement
    state_correction = state_prediction + Kalman_Gain*(Z - H*state_prediction); %4x1 vector of states

    %compute covariance correction
    covariance_correction = (eye(2) - Kalman_Gain*H)*covariance_prediction; %2x2 covariance matrix

%     corrected_angle_measure = state_correction(1) - Ts*state_correction(2);
end

== matlab function Free_Flight_PID_RPY_ARDrone_TrayZ/Navigation System/Kalman Filter/Ultrasound Estimator/Kalman Tracker ==
  data: UltraSoundMeasure input; state_correction output; covariance_correction output; covariance_correction_input input; state_correction_input input
function [state_correction, covariance_correction] = fcn(UltraSoundMeasure, covariance_correction_input,state_correction_input)


%-------------------------------
%-------------------------------
%---- Predict Stage ------------
%-------------------------------
%-------------------------------

%our states:
%  [Wx Wy Wz Bx By Bz   ]
%

p_var = 1e-2;
Ts = 1/400;
%Process Noise

Q = [p_var^2     0     
      0         p_var^2 ];

%A matrix
A =  [1   Ts    
      0   1];

%odutput these values with a unit delay (for algebraic loop), apply initial conditions
state_prediction = A*state_correction_input;
covariance_prediction_ = A*covariance_correction_input*A' + Q;

%-------------------------------
%-------------------------------
%---- Estimate Stage -----------
%-------------------------------
%-------------------------------
    %H matrix
    H = [1 0];

    %Measurement noise
    m_var = 1;
%     m_var_r = 1;

    R = [m_var^2];

    %Measurement Z
    Z = UltraSoundMeasure;

    %Compute Kalman Gain
    Kalman_Gain = covariance_prediction_*H'*inv(H*covariance_prediction_*H'+R); %2x2 matrix

    %compute state space correction based on measurement
    state_correction = state_prediction + Kalman_Gain*(Z - H*state_prediction); %2x1 vector of states

    %compute covariance correction
    covariance_correction = (eye(2) - Kalman_Gain*H)*covariance_prediction_; %2x2 covariance matrix

end
